simulink model "SARv2"  (R2016a)
settings: Solver=VariableStepAuto  StartTime=0.0  StopTime=.1  RelTol=1e-3
libraries: simulink x1, dspsigops x1
settings Model: Creator=ucagu  LastModifiedBy=ucagu

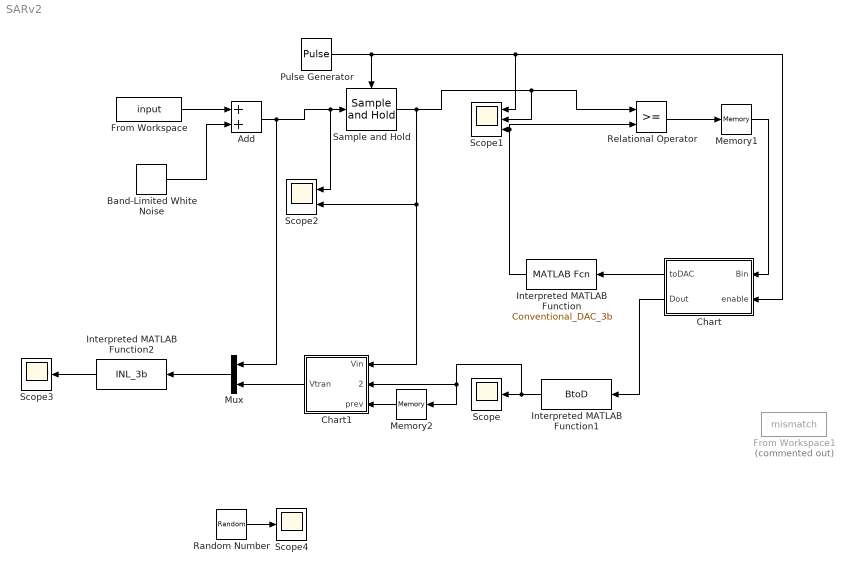
== system SARv2 ==
  Add : Sum
  Band-Limited White Noise : simulink/Sources/Band-Limited White Noise  Cov=0  Ts=1e-4  seed=[23341]
  Chart : Stateflow chart  TreatAsAtomicUnit=on
  Chart1 : Stateflow chart  TreatAsAtomicUnit=on
  From Workspace : FromWorkspace  VariableName=input  SampleTime=1e-4
  From Workspace1 : FromWorkspace  Commented=on  VariableName=mismatch  SampleTime=0
  Interpreted MATLAB Function : MATLABFcn  MATLABFcn=Conventional_DAC_3b
  Interpreted MATLAB Function1 : MATLABFcn  MATLABFcn=BtoD
  Interpreted MATLAB Function2 : MATLABFcn  MATLABFcn=INL_3b
  Memory1 : Memory  InheritSampleTime=on  LinearizeAsDelay=on
  Memory2 : Memory  InheritSampleTime=on  LinearizeAsDelay=on
  Mux : Mux  Inputs=2
  Pulse Generator : DiscretePulseGenerator  PulseType=Time based  Period=.002  PulseWidth=50
  Random Number : RandomNumber  SampleTime=0.01
  Relational Operator : RelationalOperator  OutDataTypeStr=boolean
  Sample and Hold : dspsigops/Sample and Hold  trig=Rising edge  initCond=0  latchinput=off
  Scope : Scope
  Scope1 : Scope  NumInputPorts=3
  Scope2 : Scope  NumInputPorts=2
  Scope3 : Scope
  Scope4 : Scope
  wires:
  Pulse Generator/1 -> Chart/2(enable), Scope1/1, Sample and Hold/Trigger
  Relational Operator/1 -> Memory1/1
  Sample and Hold/1 -> Chart1/1(Vin), Scope2/2, Scope1/2, Relational Operator/1
  From Workspace/1 -> Add/1
  Add/1 -> Mux/1, Scope2/1, Sample and Hold/1
  Band-Limited White Noise/1 -> Add/2
  Interpreted MATLAB Function/1 -> Scope1/3, Relational Operator/2
  Chart/1(toDAC) -> Interpreted MATLAB Function/1
  Memory1/1 -> Chart/1(Bin)
  Chart/2(Dout) -> Interpreted MATLAB Function1/1
  Interpreted MATLAB Function1/1 -> Chart1/2(current), Memory2/1, Scope/1
  Memory2/1 -> Chart1/3(prev)
  Interpreted MATLAB Function2/1 -> Scope3/1
  Mux/1 -> Interpreted MATLAB Function2/1
  Chart1/1(Vtran) -> Mux/2
  Random Number/1 -> Scope4/1

== stateflow chart SARv2/Chart1 ==
  state wait
  state tran
    entry: Vtran = Vin;
  (default) -> wait
  wait -> tran : [current > prev]
  tran -> wait : [current == prev]
  data: Vin input; current input; prev input; Vtran output

== stateflow chart SARv2/Chart ==
  state B4
    entry: Bout(3) = 1;
    entry: toDAC = Bout;
  state B6
    entry: Bout(3) = 1;
    entry: Dout = Bout;
  state B2
    entry: Bout(2) = 1;
    entry: toDAC = Bout;
  state B1
    entry: toDAC = [1 0 0 ];
    entry: Bout =[1 0 0];
  state B5
    entry: Bout(3) = 1;
    entry: Bout(2) = 0;
    entry: toDAC = Bout;
  state B7
    entry: Bout(3) = 0;
    entry: Dout = Bout;
  state B3
    entry: Bout(2) = 1;
    entry: Bout(1) = 0;
    entry: toDAC = Bout;
  B6 -> B1 : [enable == 1]
  B1 -> B2 [order 2] : [Bin==1& enable ==0]
  B2 -> B4 [order 2] : [Bin==1]
  B4 -> B6 [order 2] : [Bin==1]
  (default) -> B1
  B2 -> B5 [order 1] : [Bin==0]
  B3 -> B4 [order 1] : [Bin==1]
  B4 -> B7 [order 1] : [Bin==0]
  B5 -> B6 [order 1] : [Bin==1]
  B7 -> B1 : [enable == 1]
  B1 -> B3 [order 1] : [Bin==0 & enable == 0]
  B5 -> B7 [order 2] : [Bin==0]
  B3 -> B5 [order 2] : [Bin==0]
  data: toDAC output; Bin input; enable input; Dout output; Bout local double
